simulink model "model"  (R2023a)
settings: Solver=VariableStepAuto  StartTime=0.0  StopTime=10.0  RelTol=1e-3
settings Model: Creator=Theomur  LastModifiedBy=Theomur

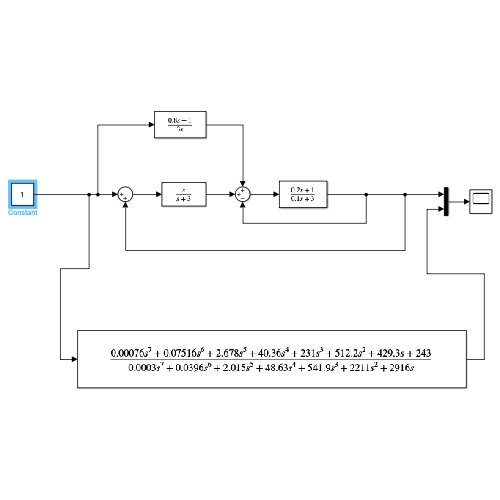
[thumbnail: Simulink's stored preview of the top-level diagram]
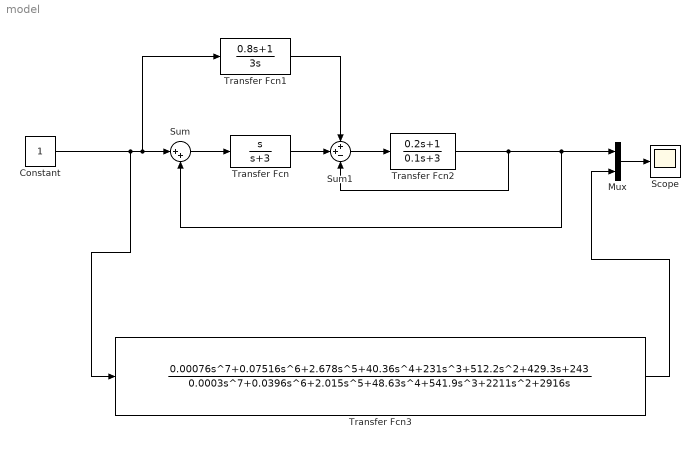
== system model ==
  Constant : Constant
  Mux : Mux  Inputs=2
  Scope : Scope
  Sum : Sum  Inputs=|++
  Sum1 : Sum  Inputs=++-
  Transfer Fcn : TransferFcn  Numerator=[1 0]  Denominator=[1 3]
  Transfer Fcn1 : TransferFcn  Numerator=[0.8 1]  Denominator=[3 0]
  Transfer Fcn2 : TransferFcn  Numerator=[0.2 1]  Denominator=[0.1 3]
  Transfer Fcn3 : TransferFcn  Numerator=[0.00076 0.07516 2.678 40.36 231 512.2 429.3 243]  Denominator=[0.0003 0.0396 2.015 48.63 541.9 2211 2916 0]
  wires:
  Constant/1 -> Transfer Fcn3/1, Transfer Fcn1/1, Sum/1
  Sum/1 -> Transfer Fcn/1
  Transfer Fcn/1 -> Sum1/2
  Sum1/1 -> Transfer Fcn2/1
  Transfer Fcn2/1 -> Sum1/3, Mux/1, Sum/2
  Transfer Fcn1/1 -> Sum1/1
  Mux/1 -> Scope/1
  Transfer Fcn3/1 -> Mux/2
